simulink model "twopulserect_inductfilter"  (R2014a)
settings: Solver=ode3  StartTime=0.0  StopTime=0.1  FixedStep=0.0001  RelTol=1e-3
libraries: fl_lib x9, nesl_utility x6, pe_lib x4
settings Model: Creator=Sergey Litvinov  LastModifiedBy=Sergey Litvinov

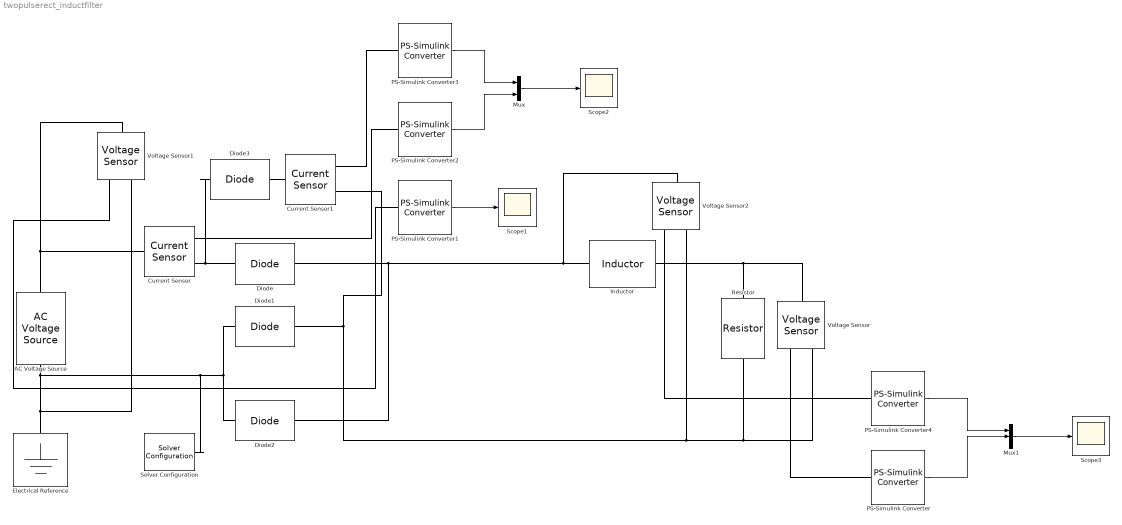
== system twopulserect_inductfilter ==
  AC Voltage Source : fl_lib/Electrical/Electrical Sources/AC Voltage Source  amp=300 V  shift=0 deg  frequency=50 Hz  omega=0 rad/s
  Current Sensor : fl_lib/Electrical/Electrical Sensors/Current Sensor
  Current Sensor1 : fl_lib/Electrical/Electrical Sensors/Current Sensor
  Diode{,1..3} (4 alike) : pe_lib/Semiconductors/Fundamental Components/Diode  Vf=0.8 V  Ron=0.001 Ohm  Goff=1e-5 1/Ohm  N_series=1  N_parallel=1  Vf_equiv=0.8 V  Ron_equiv=0.001 Ohm  Goff_equiv=1e-5 1/Ohm
  Electrical Reference : fl_lib/Electrical/Electrical Elements/Electrical Reference
  Inductor : fl_lib/Electrical/Electrical Elements/Inductor  l=1 H  r=0 Ohm  g=1e-9 1/Ohm  i_specify=off  i_priority=High  i=0 A  v_specify=off  v_priority=High  v=0 V  i_L_specify=off  i_L_priority=High  i_L=0 A
  Mux : Mux  Inputs=2
  Mux1 : Mux  Inputs=3
  PS-Simulink Converter{,1..4} (5 alike) : nesl_utility/PS-Simulink Converter  PhysicalDomain=network_engine_domain  SubClassName=ps_output  LeftPortType=input  RightPortType=output  PseudoPeriodic=off  Frequencies=[]  Unit=1  AffineConversion=off
  Resistor : fl_lib/Electrical/Electrical Elements/Resistor  R=600 Ohm  i_specify=off  i_priority=High  i=0 A  v_specify=off  v_priority=High  v=0 V
  Scope1 : Scope
  Scope2 : Scope
      settings: SaveName=ScopeData2
  Scope3 : Scope
  Solver Configuration : nesl_utility/Solver Configuration  PhysicalDomain=network_engine_domain  SubClassName=solver  LeftPortType=input  RightPortType=generic  Accelerate=off  Tones=[]  Harmonics=[]  SimulateNoise=off  Profile=off  UseLocalSampling=off  EnableSwitchedLinearOptims=on  FrequencyDomain=off  UseCCode=off  RelTol=0.001  AbsTol=1e-06  MinStep=1e-09  ToWorkspace=off  DoDC=off  ResidualTolerance=1e-09  UseLocalSolver=off  LocalSolverChoice=NE_BACKWARD_EULER_ADVANCER  LocalSolverSampleTime=0.001  DoFixedCost=off  MaxNonlinIter=3  MaxModeIter=2  LinearAlgebra=Sparse  DelaysMemoryBudget=1024  AutomaticFiltering=on  FilteringTimeConstant=0.001
  Voltage Sensor : fl_lib/Electrical/Electrical Sensors/Voltage Sensor
  Voltage Sensor1 : fl_lib/Electrical/Electrical Sensors/Voltage Sensor
  Voltage Sensor2 : fl_lib/Electrical/Electrical Sensors/Voltage Sensor
  wires:
  PS-Simulink Converter1/1 -> Scope1/1
  Mux/1 -> Scope2/1
  PS-Simulink Converter3/1 -> Mux/1
  PS-Simulink Converter2/1 -> Mux/2
  PS-Simulink Converter4/1 -> Mux1/1
  PS-Simulink Converter/1 -> Mux1/2
  Mux1/1 -> Scope3/1
  connections:
  AC Voltage Source/RConn1 -- Solver Configuration/RConn1 -- Diode2/LConn1 -- Diode1/RConn1 -- Voltage Sensor1/RConn2 -- Electrical Reference/LConn1
  Current Sensor/RConn2 -- Diode3/RConn1 -- Diode/LConn1
  Diode/RConn1 -- Voltage Sensor2/LConn1 -- Inductor/LConn1 -- Diode2/RConn1
  Voltage Sensor1/LConn1 -- AC Voltage Source/LConn1 -- Current Sensor/LConn1
  Diode3/LConn1 -- Current Sensor1/LConn1
  Current Sensor1/RConn1 -- PS-Simulink Converter3/LConn1
  Voltage Sensor/RConn1 -- PS-Simulink Converter/LConn1
  Voltage Sensor1/RConn1 -- PS-Simulink Converter1/LConn1
  Current Sensor/RConn1 -- PS-Simulink Converter2/LConn1
  Diode1/LConn1 -- Resistor/RConn1 -- Voltage Sensor/RConn2 -- Voltage Sensor2/RConn2 -- Current Sensor1/RConn2
  Resistor/LConn1 -- Voltage Sensor/LConn1 -- Inductor/RConn1
  Voltage Sensor2/RConn1 -- PS-Simulink Converter4/LConn1
